simulink model "inverterfedmotor"  (Simulink 10.0)
settings: Solver=ode45  StartTime=0.0  StopTime=10.0  RelTol=1e-3  EnableMultiTasking=on
libraries: powerlib x23, powerlib_extras x1, simulink x1
settings Model: Creator=lenovo  LastModifiedBy=asuresh4
settings DataIOCC: LimitDataPoints=on  SignalLoggingSaveFormat=ModelDataLogs
settings OptimizationCC: ExpressionDepthLimit=2147483647
settings DebuggingCC: SolverPrmCheckMsg=warning  FcnCallInpInsideContextMsg=warning  StateNameClashWarn=warning
settings ConfigComp: CovExternalEMLEnable=off

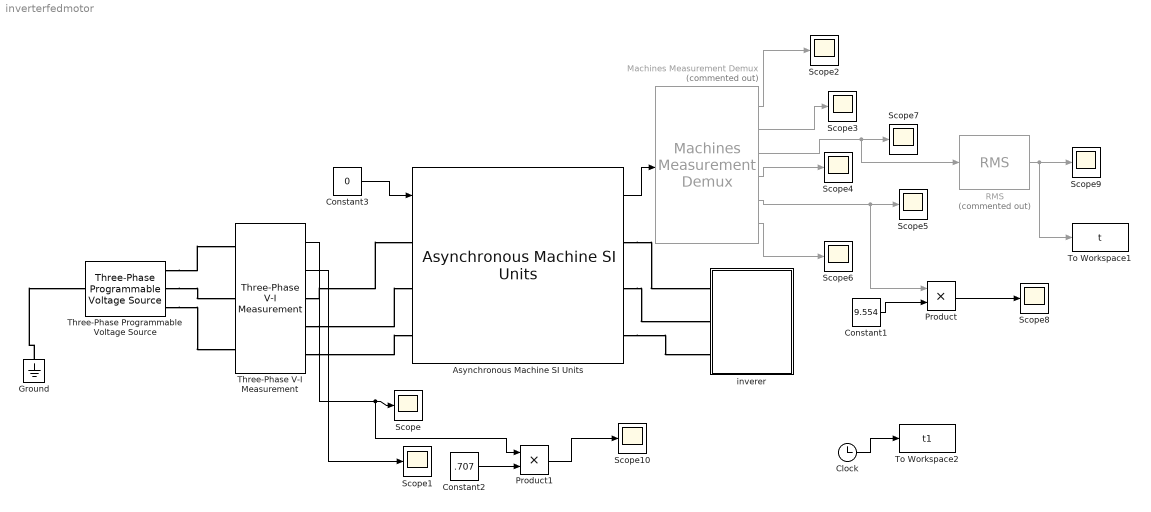
== system inverterfedmotor ==
  Asynchronous Machine SI Units : powerlib/Machines/Asynchronous Machine SI Units  RotorType=Wound  PresetModel=No  MechanicalLoad=Torque Tm  ShowDetailedParameters=on  ReferenceFrame=Synchronous  Units=SI  MeasurementBus=off  NominalParameters=[ 5*746, 415, 50 ]  Stator=[2.53 0.027]  Rotor=[ 4.692 0.027]  Cage1=[0.4155 0.002066]  Cage2=[0.4168 0.0003495]  Lm=2.308  Mechanical="[ 0.102 0  2 ]"  PolePairs=2  InitialConditions=[1 0 0 0 0 0 0 0]  SimulateSaturation=off  Saturation=[14.03593122, 27.81365428, 53.79336849, 72.68890987, 97.98006896, 148.6815601, 215.7428561, 302.9841135, 428.7778367 ; 230, 322, 414, 460, 506, 552, 598, 644, 690]  LoadFlowParameters=1492000  TsPowergui=0  TsBlock=-1  IterativeModel=Forward Euler  IterativeDiscreteModel=Trapezoidal non iterative  Pmec=1.492e+006
      settings: SourceProductName=Simscape Electrical
  Clock : Clock
  Constant1 : Constant  Value=9.554
  Constant2 : Constant  Value=.707
  Constant3 : Constant  Value=0
  Ground : powerlib/Elements/Ground  LConnTagsString=a
      settings: SourceProductName=Simscape Electrical
  Machines Measurement Demux : powerlib/Machines/Machines Measurement Demux  Commented=on  SystemSampleTime=-1  machType=Asynchronous  ssm1=on  ssm2=on  ssm3=on  ssm4=on  ssm5=on  ssm6=on  sm1=off  sm2=off  sm3=off  sm4=off  sm5=off  sm6=off  sm7=off  sm8=on  sm9=off  sm10=off  sm11=off  sm115=off  sm12=off  sm13=off  sm14=off  asm1=on  asm2=off  asm3=off  asm4=on  asm5=on  asm6=off  asm7=off  asm8=on  asm9=on  asm10=on  asm11=off  pmsm1=on  pmsm2=on  pmsm3=on  pmsm4=off  pmsm5=on  pmsm6=on  pmsm7=on  lastType=1
      settings: SourceProductName=Simscape Electrical  SourceProductBaseCode=PS
  Product : Product  RndMeth=Zero
  Product1 : Product  RndMeth=Zero
  RMS : powerlib_extras/Measurements/RMS  Commented=on  f1=60
      settings: SourceProductName=Simscape Electrical  SourceProductBaseCode=PS
  Scope{,1..10} (11 alike) : Scope
  Three-Phase Programmable Voltage Source : powerlib/Electrical Sources/Three-Phase Programmable Voltage Source  PositiveSequence=[415 0 50]  VariationEntity=None  VariationType=Step  VariationTypeAlt=Step  VariationStep=0.5  VariationRate=10  VariationMagnitude=0.3  VariationFrequency=2  VariationTiming=[1 2]  VariationPhaseA=off  Amplitudes=[1 0.8 1.2 1.0]  TimeValues=[0 0.1 0.15 0.2]  HarmonicGeneration=off  HarmonicA=[3 0.2 -25 0]  HarmonicB=[2 0.15 35 2]  Timing="[0.05  3]"  BusType=swing  Pref=0  Qref=0  Qmin=-inf  Qmax=inf
      settings: SourceProductName=Simscape Electrical
  Three-Phase V-I Measurement : powerlib/Measurements/Three-Phase V-I Measurement  VoltageMeasurement=phase-to-phase  SetLabelV=off  LabelV=Vabc  Vpu=off  VpuLL=off  CurrentMeasurement=yes  SetLabelI=off  LabelI=Iabc  Ipu=off  Pbase=100e6  Vbase=500e3  OutputType=Complex  PhasorSimulation=off  PSBequivalent=0
      settings: SourceProductName=Simscape Electrical
  To Workspace1 : ToWorkspace  VariableName=t  SampleTime=1
  To Workspace2 : ToWorkspace  VariableName=t1  SampleTime=1
  inverer : Subsystem
  wires:
  Asynchronous Machine SI Units/1 -> Machines Measurement Demux/1
  Three-Phase V-I Measurement/1 -> Scope/1, Product1/1
  Three-Phase V-I Measurement/2 -> Scope1/1
  Machines Measurement Demux/1 -> Scope2/1
  Machines Measurement Demux/2 -> Scope3/1
  Machines Measurement Demux/5 -> Scope5/1, Product/1
  Machines Measurement Demux/6 -> Scope6/1
  Machines Measurement Demux/4 -> Scope4/1
  Machines Measurement Demux/3 -> Scope7/1, RMS/1
  Constant1/1 -> Product/2
  Product/1 -> Scope8/1
  RMS/1 -> Scope9/1, To Workspace1/1
  Constant2/1 -> Product1/2
  Product1/1 -> Scope10/1
  Constant3/1 -> Asynchronous Machine SI Units/1
  Clock/1 -> To Workspace2/1
  connections:
  Three-Phase Programmable Voltage Source/RConn2 -- Three-Phase V-I Measurement/LConn2
  Ground/LConn1 -- Three-Phase Programmable Voltage Source/LConn1
  Three-Phase Programmable Voltage Source/RConn1 -- Three-Phase V-I Measurement/LConn1
  Three-Phase V-I Measurement/RConn3 -- Asynchronous Machine SI Units/LConn3
  Three-Phase V-I Measurement/RConn2 -- Asynchronous Machine SI Units/LConn2
  Three-Phase Programmable Voltage Source/RConn3 -- Three-Phase V-I Measurement/LConn3
  Three-Phase V-I Measurement/RConn1 -- Asynchronous Machine SI Units/LConn1
  Asynchronous Machine SI Units/RConn1 -- inverer/LConn1
  Asynchronous Machine SI Units/RConn2 -- inverer/LConn2
  Asynchronous Machine SI Units/RConn3 -- inverer/LConn3

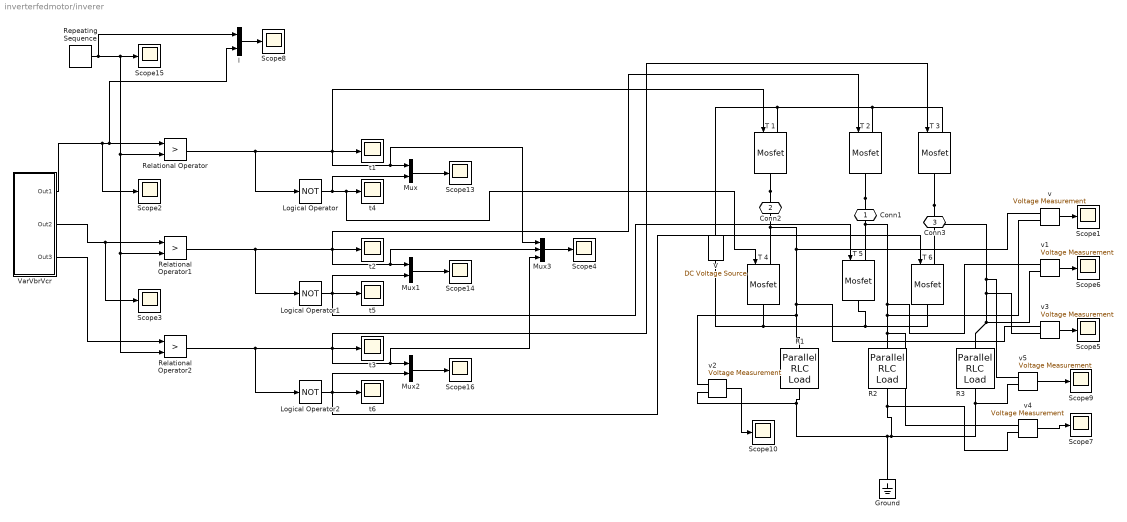
== system inverterfedmotor/inverer ==
  "     R2" : powerlib/Elements/Parallel RLC Load  LConnTagsString=a  RConnTagsString=__new0  NominalVoltage=1000  NominalFrequency=50  ActivePower=10e3  InductivePower=0  CapacitivePower=0  Setx0=off  InitialVoltage=0  SetiL0=off  InitialCurrent=0  Measurements=None  LoadType=constant Z
      settings: AttributesFormatString=\n  SourceProductName=Simscape Electrical  SourceProductBaseCode=PS
  Ground : powerlib/Elements/Ground  LConnTagsString=a
      settings: SourceProductName=Simscape Electrical
  Logical Operator : Logic  Operator=NOT  AllPortsSameDT=off  OutDataTypeStr=boolean
  Logical Operator1 : Logic  Operator=NOT  AllPortsSameDT=off  OutDataTypeStr=boolean
  Logical Operator2 : Logic  Operator=NOT  AllPortsSameDT=off  OutDataTypeStr=boolean
  Mux : Mux  Inputs=2
  Mux1 : Mux  Inputs=2
  Mux2 : Mux  Inputs=2
  Mux3 : Mux  Inputs=3
  R1 : powerlib/Elements/Parallel RLC Load  LConnTagsString=a  RConnTagsString=__new0  NominalVoltage=1000  NominalFrequency=50  ActivePower=10e3  InductivePower=0  CapacitivePower=0  Setx0=off  InitialVoltage=0  SetiL0=off  InitialCurrent=0  Measurements=Branch voltage  LoadType=constant Z
      settings: AttributesFormatString=\n  SourceProductName=Simscape Electrical  SourceProductBaseCode=PS
  R3 : powerlib/Elements/Parallel RLC Load  LConnTagsString=a  RConnTagsString=__new0  NominalVoltage=1000  NominalFrequency=50  ActivePower=10e3  InductivePower=0  CapacitivePower=0  Setx0=off  InitialVoltage=0  SetiL0=off  InitialCurrent=0  Measurements=None  LoadType=constant Z
      settings: AttributesFormatString=\n  SourceProductName=Simscape Electrical  SourceProductBaseCode=PS
  Relational Operator : RelationalOperator  Operator=>  OutDataTypeStr=boolean  RndMeth=Nearest
  Relational Operator1 : RelationalOperator  Operator=>  OutDataTypeStr=boolean  RndMeth=Nearest
  Relational Operator2 : RelationalOperator  Operator=>  OutDataTypeStr=boolean  RndMeth=Nearest
  Repeating Sequence : simulink/Sources/Repeating Sequence  rep_seq_t=[0 0.1 0.2 0.3 0.4 0.5 0.6 0.7 0.8 0.9 1 1.1 1.2 1.3 1.4 1.5 1.6 1.7 1.8]  rep_seq_y=[1 -1 1 -1 1 -1 1 -1 1 -1 1 -1 1 -1 1 -1 1 -1 1]
  Scope{1..10,13..16} (14 alike) : Scope
  T {1..6} (6 alike) : powerlib/Power Electronics/Mosfet  Ron=0.1  Lon=0  Rd=0.01  Vfd=0  IC=0  Rs=1e5  Cs=inf  Measurements=off
      settings: SourceProductName=Simscape Electrical
  V : powerlib/Electrical Sources/DC Voltage Source  Amplitude=300  Measurements=Voltage
      settings: SourceProductName=Simscape Electrical
  VarVbrVcr : Subsystem
  l : Concatenate
  t{1..6} (6 alike) : Scope
  v{,1..5} (6 alike) : powerlib/Measurements/Voltage Measurement  PhasorSimulation=off  OutputType=Complex  PSBequivalent=0
      settings: SourceProductName=Simscape Electrical
  Conn1 : PMIOPort  Side=Left
  Conn2 : PMIOPort  Port=2  Side=Left
  Conn3 : PMIOPort  Port=3  Side=Left
  wires:
  VarVbrVcr/2(Out2) -> Relational Operator1/1, Scope3/1
  VarVbrVcr/3(Out3) -> Relational Operator2/1
  Relational Operator/1 -> Logical Operator/1, t1/1, Mux/1, Mux3/1, T 1/1
  Relational Operator1/1 -> Logical Operator1/1, t2/1, Mux1/1, Mux3/2, T 2/1
  Relational Operator2/1 -> Logical Operator2/1, t3/1, Mux2/1, Mux3/3, T 3/1
  Logical Operator/1 -> Mux/2, t4/1, T 4/1
  Logical Operator1/1 -> Mux1/2, T 5/1, t5/1
  Logical Operator2/1 -> t6/1, T 6/1, Mux2/2
  Mux1/1 -> Scope14/1
  Mux2/1 -> Scope16/1
  Mux/1 -> Scope13/1
  Repeating Sequence/1 -> Relational Operator/2, Relational Operator2/2, Relational Operator1/2, Scope15/1, l/1
  Mux3/1 -> Scope4/1
  v/1 -> Scope1/1
  v1/1 -> Scope6/1
  v3/1 -> Scope5/1
  v2/1 -> Scope10/1
  v4/1 -> Scope7/1
  v5/1 -> Scope9/1
  l/1 -> Scope8/1
  VarVbrVcr/1(Out1) -> Scope2/1, Relational Operator/1, l/2
  connections:
  T 5/LConn1 -- v4/LConn1 -- "     R2"/LConn1 -- v/LConn2 -- v1/LConn1 -- T 2/RConn1 -- Conn1/RConn1
  R3/RConn1 -- v5/LConn2 -- Ground/LConn1 -- R1/RConn1 -- v2/LConn2 -- "     R2"/RConn1 -- v4/LConn2
  R1/LConn1 -- v3/LConn1 -- T 4/LConn1 -- T 1/RConn1 -- Conn2/RConn1 -- v/LConn1 -- v2/LConn1
  v5/LConn1 -- T 6/LConn1 -- T 3/RConn1 -- Conn3/RConn1 -- v3/LConn2 -- R3/LConn1 -- v1/LConn2
  T 3/LConn1 -- T 2/LConn1 -- T 1/LConn1 -- V/RConn1
  T 6/RConn1 -- T 4/RConn1 -- V/LConn1 -- T 5/RConn1

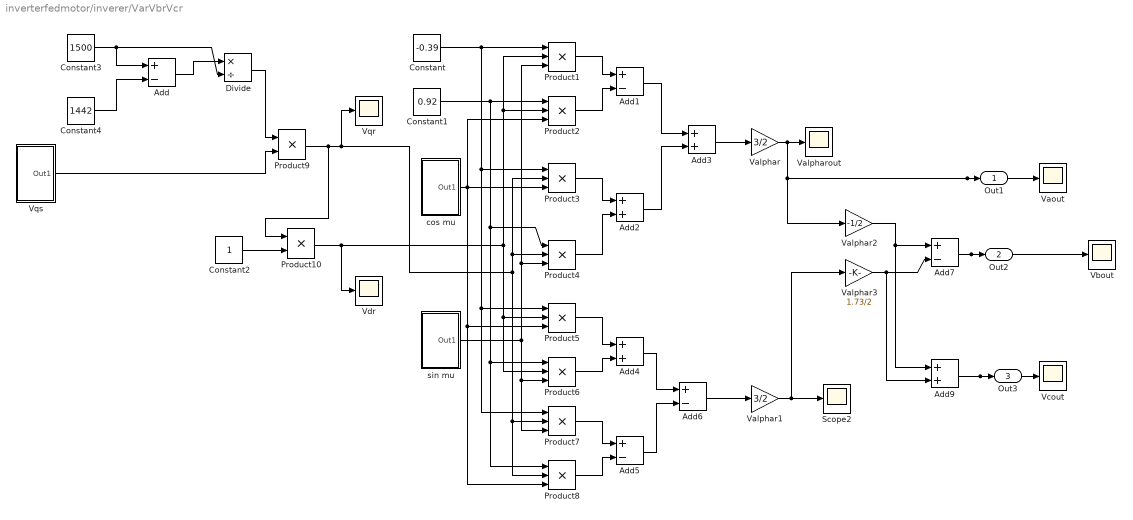
== system inverterfedmotor/inverer/VarVbrVcr ==
  Add{,1,5..7} (5 alike) : Sum  Inputs=+-
  Add{2..4,9} (4 alike) : Sum
  Constant : Constant  Value=-0.39
  Constant1 : Constant  Value=0.92
  Constant2 : Constant
  Constant3 : Constant  Value=1500
  Constant4 : Constant  Value=1442
  Divide : Product  Inputs=*/
  Product{1..8} (8 alike) : Product  Inputs=3  RndMeth=Zero
  Product10 : Product  RndMeth=Zero
  Product9 : Product  RndMeth=Zero
  Scope2 : Scope
  Valphar : Gain  Gain=3/2
  Valphar1 : Gain  Gain=3/2
  Valphar2 : Gain  Gain=-1/2
  Valphar3 : Gain  Gain=1.73/2
  Valpharout : Scope
  Vaout : Scope
  Vbout : Scope
  Vcout : Scope
  Vdr : Scope
  Vqr : Scope
  Vqs : Subsystem
  cos mu : Subsystem
  sin mu : Subsystem
  Out1 : Outport
  Out2 : Outport  Port=2
  Out3 : Outport  Port=3
  wires:
  Constant/1 -> Product1/1, Product3/1, Product5/1, Product7/1
  sin mu/1(Out1) -> Product1/3, Product4/3, Product6/3, Product7/3
  Constant1/1 -> Product2/1, Product4/1, Product6/1, Product8/1
  cos mu/1(Out1) -> Product3/3, Product2/3, Product5/3, Product8/3
  Product1/1 -> Add1/1
  Product2/1 -> Add1/2
  Product3/1 -> Add2/1
  Product4/1 -> Add2/2
  Add1/1 -> Add3/1
  Add2/1 -> Add3/2
  Add3/1 -> Valphar/1
  Valphar/1 -> Valphar2/1, Vaout/1, Out1/1, Valpharout/1
  Valphar1/1 -> Scope2/1, Valphar3/1
  Add6/1 -> Valphar1/1
  Add4/1 -> Add6/1
  Add5/1 -> Add6/2
  Product5/1 -> Add4/1
  Product6/1 -> Add4/2
  Product7/1 -> Add5/1
  Product8/1 -> Add5/2
  Add7/1 -> Vbout/1, Out2/1
  Valphar3/1 -> Add7/2, Add9/2
  Valphar2/1 -> Add7/1, Add9/1
  Add9/1 -> Vcout/1, Out3/1
  Constant3/1 -> Add/1, Divide/2
  Constant4/1 -> Add/2
  Add/1 -> Divide/1
  Divide/1 -> Product9/1
  Constant2/1 -> Product10/2
  Product9/1 -> Product10/1, Vqr/1, Product3/2, Product4/2, Product7/2, Product8/2
  Product10/1 -> Vdr/1, Product1/2, Product2/2, Product5/2, Product6/2
  Vqs/1(Out1) -> Product9/2

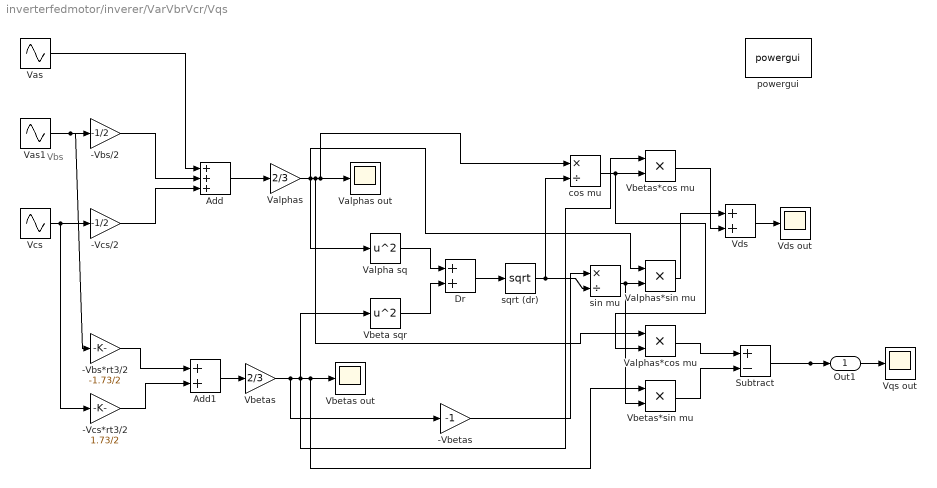
== system inverterfedmotor/inverer/VarVbrVcr/Vqs ==
  note: Vbs
  "-Vbetas " : Gain  Gain=-1
  -Vbs*rt3/2 : Gain  Gain=-1.73/2
  -Vbs/2 : Gain  Gain=-1/2
  -Vcs*rt3/2 : Gain  Gain=1.73/2
  -Vcs/2 : Gain  Gain=-1/2
  Add : Sum  Inputs=+++
  Add1 : Sum
  Dr : Sum
  Subtract : Sum  Inputs=+-
  Valpha sq : Math  Operator=square  SaturateOnIntegerOverflow=on
  Valphas : Gain  Gain=2/3
  Valphas out : Scope
  Valphas*cos mu : Product  RndMeth=Zero
  Valphas*sin mu : Product  RndMeth=Zero
  Vas : Sin  Amplitude=230  Frequency=314  SampleTime=0
  Vas1 : Sin  Amplitude=230  Frequency=314  Phase=-2.09  SampleTime=0
  Vbeta sqr : Math  Operator=square  SaturateOnIntegerOverflow=on
  Vbetas : Gain  Gain=2/3
  Vbetas out : Scope
  Vbetas*cos mu : Product  RndMeth=Zero
  Vbetas*sin mu : Product  RndMeth=Zero
  Vcs : Sin  Amplitude=230  Frequency=314  Phase=-4.18  SampleTime=0
  Vds : Sum
  Vds out : Scope
  Vqs out : Scope
  cos mu : Product  Inputs=*/
  powergui : powerlib/powergui  Priority=1  SimulationMode=Continuous  SampleTime=50e-6  frequency=60  Iterations=50  frequencyindice=50  Pbase=100e6  ErrMax=1e-4  UnitsV=kV  UnitsW=MW  buscounter=0  FunctionMessages=off  echomessages=off  EnableUseOfTLC=off  CurrentSourceSwitches=off  DisableSnubberDevices=off  DisableRonSwitches=off  DisableVfSwitches=off  DisplayEquations=off  AutomaticDiscreteSolvers=off  SolverType=Tustin/Backward Euler (TBE)  Interpol=off  ExternalGateDelay=off  methode=off  Ts=0  x0status=blocks  SPID=off  SwTol=0  HookPort=off  NonlinearTolerance=1e-4  nMaxIteration=100  ContinueOnMaxIteration=off  RestoreLinks=warning  ResistiveCurrentMeasurement=off  Frange=[0:2:500]  Ylog=off  Xlog=on  ShowGrid=off  save=off  variable=ZData  structure=0  ZoomFFT=on  StartTime=0.0  cycles=1  DisplayStyle=1  fundamental=60  FreqAxis=off  MaxFrequency=1000  frequencyindicesteady=1  RmsSteady=1  display=off
      settings: SourceProductName=Simscape Electrical
  sin mu : Product  Inputs=*/
  sqrt (dr) : Math  Operator=sqrt  SaturateOnIntegerOverflow=on
  Out1 : Outport
  wires:
  Vas1/1 -> -Vbs/2/1, -Vbs*rt3/2/1
  Vcs/1 -> -Vcs/2/1, -Vcs*rt3/2/1
  Vas/1 -> Add/1
  -Vbs/2/1 -> Add/2
  -Vcs/2/1 -> Add/3
  Add/1 -> Valphas/1
  -Vbs*rt3/2/1 -> Add1/1
  -Vcs*rt3/2/1 -> Add1/2
  Add1/1 -> Vbetas/1
  Valphas/1 -> Valpha sq/1, Valphas*sin mu/1, Valphas out/1, cos mu/1, Valphas*cos mu/1
  Vbetas/1 -> Vbeta sqr/1, Vbetas*cos mu/1, Vbetas out/1, Vbetas*sin mu/1, "-Vbetas "/1
  Valpha sq/1 -> Dr/1
  Vbeta sqr/1 -> Dr/2
  Dr/1 -> sqrt (dr)/1
  "-Vbetas "/1 -> sin mu/1
  sqrt (dr)/1 -> sin mu/2, cos mu/2
  sin mu/1 -> Valphas*sin mu/2, Vbetas*sin mu/2
  cos mu/1 -> Vbetas*cos mu/2, Valphas*cos mu/2
  Valphas*sin mu/1 -> Vds/1
  Vbetas*cos mu/1 -> Vds/2
  Valphas*cos mu/1 -> Subtract/1
  Subtract/1 -> Vqs out/1, Out1/1
  Vbetas*sin mu/1 -> Subtract/2
  Vds/1 -> Vds out/1

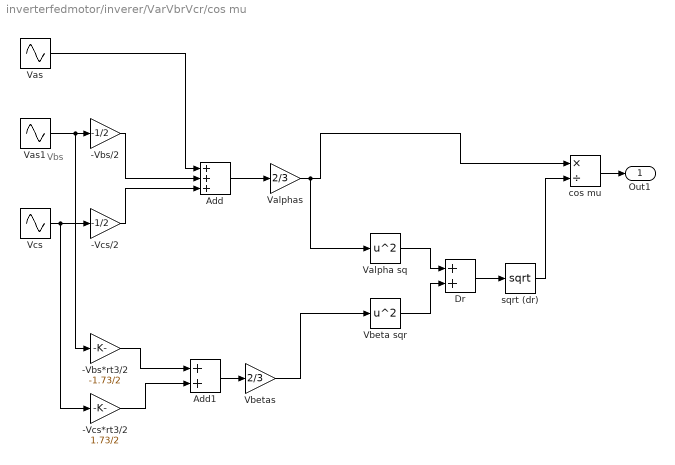
== system inverterfedmotor/inverer/VarVbrVcr/cos mu ==
  note: Vbs
  -Vbs*rt3/2 : Gain  Gain=-1.73/2
  -Vbs/2 : Gain  Gain=-1/2
  -Vcs*rt3/2 : Gain  Gain=1.73/2
  -Vcs/2 : Gain  Gain=-1/2
  Add : Sum  Inputs=+++
  Add1 : Sum
  Dr : Sum
  Valpha sq : Math  Operator=square  SaturateOnIntegerOverflow=on
  Valphas : Gain  Gain=2/3
  Vas : Sin  Amplitude=230  Frequency=314  SampleTime=0
  Vas1 : Sin  Amplitude=230  Frequency=314  Phase=-2.09  SampleTime=0
  Vbeta sqr : Math  Operator=square  SaturateOnIntegerOverflow=on
  Vbetas : Gain  Gain=2/3
  Vcs : Sin  Amplitude=230  Frequency=314  Phase=-4.18  SampleTime=0
  cos mu : Product  Inputs=*/
  sqrt (dr) : Math  Operator=sqrt  SaturateOnIntegerOverflow=on
  Out1 : Outport
  wires:
  Vas1/1 -> -Vbs/2/1, -Vbs*rt3/2/1
  Vcs/1 -> -Vcs/2/1, -Vcs*rt3/2/1
  Vas/1 -> Add/1
  -Vbs/2/1 -> Add/2
  -Vcs/2/1 -> Add/3
  Add/1 -> Valphas/1
  -Vbs*rt3/2/1 -> Add1/1
  -Vcs*rt3/2/1 -> Add1/2
  Add1/1 -> Vbetas/1
  Valphas/1 -> Valpha sq/1, cos mu/1
  Vbetas/1 -> Vbeta sqr/1
  Valpha sq/1 -> Dr/1
  Vbeta sqr/1 -> Dr/2
  Dr/1 -> sqrt (dr)/1
  sqrt (dr)/1 -> cos mu/2
  cos mu/1 -> Out1/1

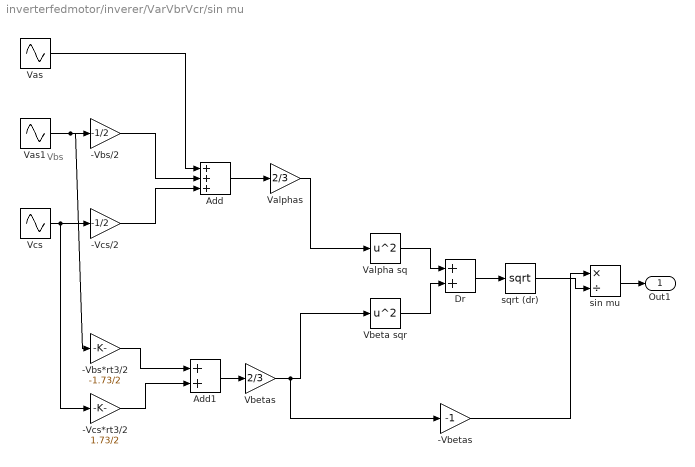
== system inverterfedmotor/inverer/VarVbrVcr/sin mu ==
  note: Vbs
  "-Vbetas " : Gain  Gain=-1
  -Vbs*rt3/2 : Gain  Gain=-1.73/2
  -Vbs/2 : Gain  Gain=-1/2
  -Vcs*rt3/2 : Gain  Gain=1.73/2
  -Vcs/2 : Gain  Gain=-1/2
  Add : Sum  Inputs=+++
  Add1 : Sum
  Dr : Sum
  Valpha sq : Math  Operator=square  SaturateOnIntegerOverflow=on
  Valphas : Gain  Gain=2/3
  Vas : Sin  Amplitude=230  Frequency=314  SampleTime=0
  Vas1 : Sin  Amplitude=230  Frequency=314  Phase=-2.09  SampleTime=0
  Vbeta sqr : Math  Operator=square  SaturateOnIntegerOverflow=on
  Vbetas : Gain  Gain=2/3
  Vcs : Sin  Amplitude=230  Frequency=314  Phase=-4.18  SampleTime=0
  sin mu : Product  Inputs=*/
  sqrt (dr) : Math  Operator=sqrt  SaturateOnIntegerOverflow=on
  Out1 : Outport
  wires:
  Vas1/1 -> -Vbs/2/1, -Vbs*rt3/2/1
  Vcs/1 -> -Vcs/2/1, -Vcs*rt3/2/1
  Vas/1 -> Add/1
  -Vbs/2/1 -> Add/2
  -Vcs/2/1 -> Add/3
  Add/1 -> Valphas/1
  -Vbs*rt3/2/1 -> Add1/1
  -Vcs*rt3/2/1 -> Add1/2
  Add1/1 -> Vbetas/1
  Valphas/1 -> Valpha sq/1
  Vbetas/1 -> "-Vbetas "/1, Vbeta sqr/1
  Valpha sq/1 -> Dr/1
  Vbeta sqr/1 -> Dr/2
  Dr/1 -> sqrt (dr)/1
  "-Vbetas "/1 -> sin mu/1
  sqrt (dr)/1 -> sin mu/2
  sin mu/1 -> Out1/1
